simulink model "manning_test_div_nonlinear"  (R2022b)
settings: Solver=VariableStepAuto  StartTime=0.0  StopTime=5*N  RelTol=1e-3
undefined symbols (not defined in the file): yd_ds
settings Model: Creator=chuan  LastModifiedBy=chuan

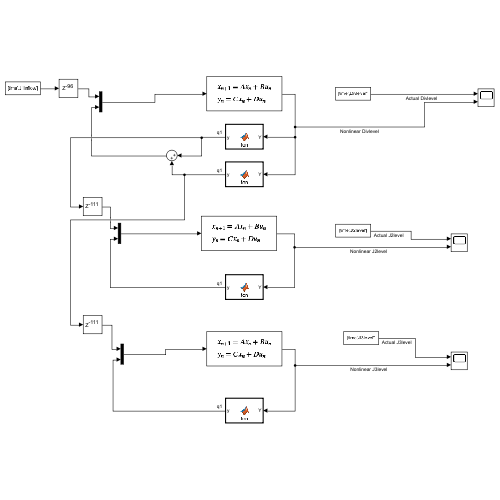
[thumbnail: Simulink's stored preview of the top-level diagram]
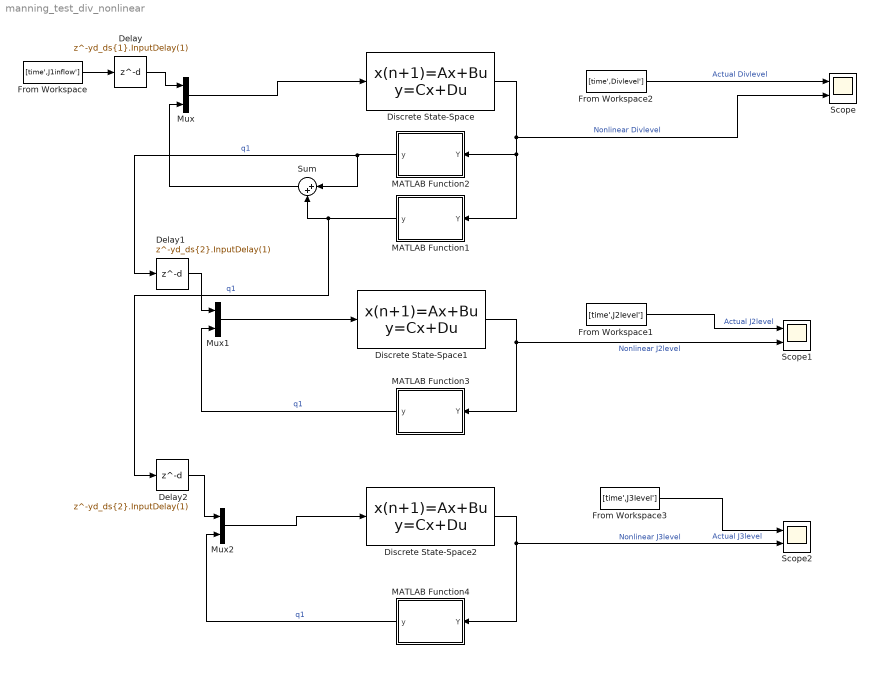
== system manning_test_div_nonlinear ==
  Delay : Delay  DelayLength=yd_ds{1}.InputDelay(1)  InitialCondition=0
  Delay1 : Delay  DelayLength=yd_ds{2}.InputDelay(1)  InitialCondition=0
  Delay2 : Delay  DelayLength=yd_ds{2}.InputDelay(1)  InitialCondition=0
  Discrete State-Space : DiscreteStateSpace  A=yd_ds{1}.A  B=yd_ds{1}.B  C=yd_ds{1}.C  D=yd_ds{1}.D  SampleTime=yd_ds{1}.Ts
  Discrete State-Space1 : DiscreteStateSpace  A=yd_ds{2}.A  B=yd_ds{2}.B  C=yd_ds{2}.C  D=yd_ds{2}.D  SampleTime=yd_ds{2}.Ts
  Discrete State-Space2 : DiscreteStateSpace  A=yd_ds{3}.A  B=yd_ds{3}.B  C=yd_ds{3}.C  D=yd_ds{3}.D  SampleTime=yd_ds{3}.Ts
  From Workspace : FromWorkspace  VariableName=[time',J1inflow']
  From Workspace1 : FromWorkspace  VariableName=[time',J2level']
  From Workspace2 : FromWorkspace  VariableName=[time',Divlevel']
  From Workspace3 : FromWorkspace  VariableName=[time',J3level']
  MATLAB Function1 : MATLAB Function  TreatAsAtomicUnit=on
  MATLAB Function2 : MATLAB Function  TreatAsAtomicUnit=on
  MATLAB Function3 : MATLAB Function  TreatAsAtomicUnit=on
  MATLAB Function4 : MATLAB Function  TreatAsAtomicUnit=on
  Mux : Mux  Inputs=2
  Mux1 : Mux  Inputs=2
  Mux2 : Mux  Inputs=2
  Scope : Scope  NumInputPorts=2
  Scope1 : Scope  NumInputPorts=2
  Scope2 : Scope  NumInputPorts=2
  Sum : Sum  Inputs=|++
  wires:
  Mux/1 -> Discrete State-Space/1
  From Workspace2/1 -> Scope/1  "Actual Divlevel"
  Discrete State-Space/1 -> Scope/2, MATLAB Function1/1(Y), MATLAB Function2/1(Y)  "Nonlinear Divlevel"
  MATLAB Function2/1(y) -> Delay1/1, Sum/1  "q1"
  MATLAB Function1/1(y) -> Sum/2, Delay2/1  "q1"
  Sum/1 -> Mux/2
  Mux1/1 -> Discrete State-Space1/1
  Discrete State-Space1/1 -> MATLAB Function3/1(Y), Scope1/2  "Nonlinear J2level"
  MATLAB Function3/1(y) -> Mux1/2  "q1"
  From Workspace1/1 -> Scope1/1  "Actual J2level"
  Mux2/1 -> Discrete State-Space2/1
  Discrete State-Space2/1 -> MATLAB Function4/1(Y), Scope2/2  "Nonlinear J3level"
  MATLAB Function4/1(y) -> Mux2/2  "q1"
  From Workspace3/1 -> Scope2/1  "Actual J3level"
  From Workspace/1 -> Delay/1
  Delay/1 -> Mux/1
  Delay1/1 -> Mux1/1
  Delay2/1 -> Mux2/1

== matlab function manning_test_div_nonlinear/MATLAB Function1 ==
  data: Y input; y output
function y = fcn(Y)
n = 0.02;
Sb = 0.0008;
B=8;
m = 1.5;

Y = max(Y,0);

y = (1/n)*(B*Y + m*Y.^2)*((B*Y + m*Y.^2)/(B + 2.*Y.*sqrt(1+m^2))).^(2/3) .* sqrt(Sb);

== matlab function manning_test_div_nonlinear/MATLAB Function2 ==
  data: Y input; y output
function y = fcn(Y)
n = 0.02;
Sb = 0.0008;
B=8;
m = 1.5;

Y = max(Y,0);

y = (1/n)*(B*Y + m*Y.^2)*((B*Y + m*Y.^2)/(B + 2.*Y.*sqrt(1+m^2))).^(2/3) .* sqrt(Sb);

== matlab function manning_test_div_nonlinear/MATLAB Function4 ==
  data: Y input; y output
function y = fcn(Y)
n = 0.02;
Sb = 0.0008;
B=8;
m = 1.5;

Y = max(Y,0);

y = (1/n)*(B*Y + m*Y.^2)*((B*Y + m*Y.^2)/(B + 2.*Y.*sqrt(1+m^2))).^(2/3) .* sqrt(Sb);

== matlab function manning_test_div_nonlinear/MATLAB Function3 ==
  data: Y input; y output
function y = fcn(Y)
n = 0.02;
Sb = 0.0008;
B=8;
m = 1.5;

Y = max(Y,0);

y = (1/n)*(B*Y + m*Y.^2)*((B*Y + m*Y.^2)/(B + 2.*Y.*sqrt(1+m^2))).^(2/3) .* sqrt(Sb);
